simulink model "v2ggg2018"  (R2018b)
settings: Solver=VariableStepAuto  StartTime=0.0  StopTime=1  RelTol=1e-3
undefined symbols (not defined in the file): Ion, Lithium
libraries: powerlib x32, electricdrivelib x1, powerlib_meascontrol x1
settings Model: Creator=user  LastModifiedBy=utkar

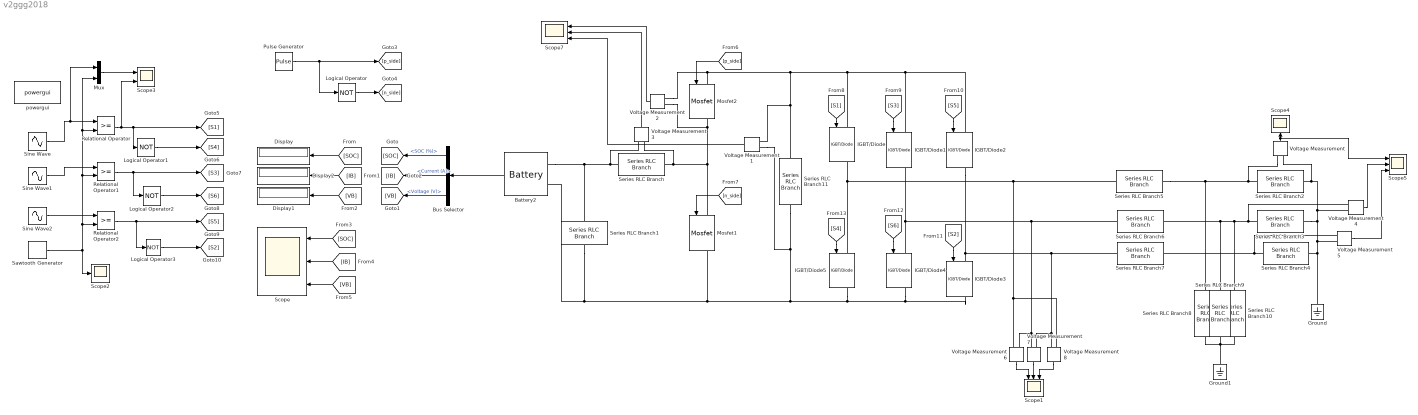
== system v2ggg2018 ==
  Battery2 : electricdrivelib/Extra Sources/Battery  BatType=Lithium-Ion  ShowTempParam=off  ThermalPreset=no  ShowAgeParam=off  NomV=24  NomQ=10  SOC=50  Batt_Tr=1e-4  PresetModel=on  MaxQ=10  MinV=18  FullV=27.9357  Dis_rate=4.3478  R=0.024  Normal_OP=9.0435  expZone="[25.9293     0.491304]"  current=[6.5 13 32.5]  Units=Time  Tci=20  NomT=20  T2=-30  MaxQ2=4.8  FullV2=7.1  Normal_OP2=5.655  expZone2="[6.58           1]"  Rca=0.6  ti=2000  Dp=0  Neq0=0  Tsim=1e6  Ta1=25  Qeol=5.4*0.9  Reol=0.013333*1.2  Char_age=[2.3478, 3]  Dis_age=[2.3478, 10]  N1=1500  N2=10500  N3=1000  N4=1400  Ta2=45  N5=950
  Bus Selector : BusSelector  OutputSignals=SOC (%),Current (A),Voltage (V)
  Display : Display
  Display1 : Display
  Display2 : Display
  Ground : powerlib/Elements/Ground  LConnTagsString=a
  Ground1 : powerlib/Elements/Ground  LConnTagsString=a
  IGBT/Diode{,1..5} (6 alike) : powerlib/Power Electronics/IGBT//Diode  Ron=1e-3  Rs=1e5  Cs=inf  Measurements=on
  Logical Operator{,1..3} (4 alike) : Logic  Operator=NOT  AllPortsSameDT=off  OutDataTypeStr=boolean
  Mosfet1 : powerlib/Power Electronics/Mosfet  Ron=0.1  Lon=0  Rd=0.01  Vfd=0  IC=0  Rs=1e5  Cs=inf  Measurements=on
  Mosfet2 : powerlib/Power Electronics/Mosfet  Ron=0.1  Lon=0  Rd=0.01  Vfd=0  IC=0  Rs=1e5  Cs=inf  Measurements=on
  Mux : Mux  Inputs=2
  Pulse Generator : DiscretePulseGenerator  PulseType=Time based  Period=1e-4  PulseWidth=40
  Relational Operator : RelationalOperator  OutDataTypeStr=boolean  RndMeth=Simplest
  Relational Operator1 : RelationalOperator  OutDataTypeStr=boolean  RndMeth=Simplest
  Relational Operator2 : RelationalOperator  OutDataTypeStr=boolean  RndMeth=Simplest
  Sawtooth Generator : powerlib_meascontrol/Pulse & Signal Generators/Sawtooth Generator  Freq=1e3  Phase=180  Ts=0
      settings: SourceProductName=Simscape Power Systems
  Scope{,1,5,7} (4 alike) : Scope  NumInputPorts=3
  Scope2 : Scope
  Scope3 : Scope  NumInputPorts=2
  Scope4 : Scope
  Series RLC Branch : powerlib/Elements/Series RLC Branch  LConnTagsString=__new0  RConnTagsString=__new0  BranchType=RL  Resistance=0.1  Inductance=1e-3  SetiL0=off  InitialCurrent=0  Capacitance=1e-6  Setx0=off  InitialVoltage=0  Measurements=None
  Series RLC Branch1 : powerlib/Elements/Series RLC Branch  LConnTagsString=__new0  RConnTagsString=__new0  BranchType=RC  Resistance=0.001  Inductance=1e-3  SetiL0=off  InitialCurrent=0  Capacitance=1000e-6  Setx0=off  InitialVoltage=0  Measurements=None
  Series RLC Branch10 : powerlib/Elements/Series RLC Branch  LConnTagsString=__new0  RConnTagsString=__new0  BranchType=C  Resistance=10  Inductance=1e-3  SetiL0=off  InitialCurrent=0  Capacitance=30e-6  Setx0=off  InitialVoltage=0  Measurements=None
  Series RLC Branch11 : powerlib/Elements/Series RLC Branch  LConnTagsString=__new0  RConnTagsString=__new0  BranchType=C  Resistance=10  Inductance=1e-3  SetiL0=off  InitialCurrent=0  Capacitance=5600e-6  Setx0=off  InitialVoltage=0  Measurements=None
  Series RLC Branch2 : powerlib/Elements/Series RLC Branch  LConnTagsString=__new0  RConnTagsString=__new0  BranchType=R  Resistance=10  Inductance=5e-3  SetiL0=off  InitialCurrent=0  Capacitance=1e-6  Setx0=off  InitialVoltage=0  Measurements=None
  Series RLC Branch3 : powerlib/Elements/Series RLC Branch  LConnTagsString=__new0  RConnTagsString=__new0  BranchType=R  Resistance=10  Inductance=5e-3  SetiL0=off  InitialCurrent=0  Capacitance=1e-6  Setx0=off  InitialVoltage=0  Measurements=None
  Series RLC Branch4 : powerlib/Elements/Series RLC Branch  LConnTagsString=__new0  RConnTagsString=__new0  BranchType=R  Resistance=10  Inductance=5e-3  SetiL0=off  InitialCurrent=0  Capacitance=1e-6  Setx0=off  InitialVoltage=0  Measurements=None
  Series RLC Branch5 : powerlib/Elements/Series RLC Branch  LConnTagsString=__new0  RConnTagsString=__new0  BranchType=L  Resistance=10  Inductance=5e-3  SetiL0=off  InitialCurrent=0  Capacitance=1e-6  Setx0=off  InitialVoltage=0  Measurements=None
  Series RLC Branch6 : powerlib/Elements/Series RLC Branch  LConnTagsString=__new0  RConnTagsString=__new0  BranchType=L  Resistance=10  Inductance=5e-3  SetiL0=off  InitialCurrent=0  Capacitance=1e-6  Setx0=off  InitialVoltage=0  Measurements=None
  Series RLC Branch7 : powerlib/Elements/Series RLC Branch  LConnTagsString=__new0  RConnTagsString=__new0  BranchType=L  Resistance=10  Inductance=5e-3  SetiL0=off  InitialCurrent=0  Capacitance=1e-6  Setx0=off  InitialVoltage=0  Measurements=None
  Series RLC Branch8 : powerlib/Elements/Series RLC Branch  LConnTagsString=__new0  RConnTagsString=__new0  BranchType=C  Resistance=10  Inductance=1e-3  SetiL0=off  InitialCurrent=0  Capacitance=30e-6  Setx0=off  InitialVoltage=0  Measurements=None
  Series RLC Branch9 : powerlib/Elements/Series RLC Branch  LConnTagsString=__new0  RConnTagsString=__new0  BranchType=C  Resistance=10  Inductance=1e-3  SetiL0=off  InitialCurrent=0  Capacitance=30e-6  Setx0=off  InitialVoltage=0  Measurements=None
  Sine Wave : Sin  Frequency=2*pi*50  SampleTime=0
  Sine Wave1 : Sin  Frequency=2*pi*50  Phase=2*pi/3  SampleTime=0
  Sine Wave2 : Sin  Frequency=2*pi*50  Phase=4*pi/3  SampleTime=0
  Voltage Measurement{,1..8} (9 alike) : powerlib/Measurements/Voltage Measurement  PhasorSimulation=off  OutputType=Complex  PSBequivalent=0
  powergui : powerlib/powergui  Priority=1  SimulationMode=Continuous  SampleTime=50e-6  frequency=60  Iterations=50  frequencyindice=0  Pbase=100e6  ErrMax=1e-4  UnitsV=kV  UnitsW=MW  buscounter=0  FunctionMessages=off  echomessages=off  EnableUseOfTLC=off  CurrentSourceSwitches=off  DisableSnubberDevices=off  DisableRonSwitches=off  DisableVfSwitches=off  DisplayEquations=off  SolverType=Tustin/Backward Euler (TBE)  Interpol=off  ExternalGateDelay=off  methode=off  Ts=100  x0status=blocks  SPID=on  SwTol=0  HookPort=off  RestoreLinks=warning  ResistiveCurrentMeasurement=off  Frange=[0:2:500]  Ylog=off  Xlog=on  ShowGrid=off  save=off  variable=ZData  structure=pasevol  ZoomFFT=off  StartTime=0.1  cycles=1  DisplayStyle=1  fundamental=50  FreqAxis=off  MaxFrequency=500  frequencyindicesteady=1  RmsSteady=1  display=off
  wires:
  Voltage Measurement3/1 -> Scope7/2
  [SOC] -> Scope/1
  [IB] -> Display2/1
  Bus Selector/2 -> [IB]  "<Current (A)>"
  Bus Selector/1 -> [SOC]  "<SOC (%)>"
  Logical Operator/1 -> [n_side]
  Bus Selector/3 -> [VB]  "<Voltage (V)>"
  [IB] -> Scope/2
  Battery2/1 -> Bus Selector/1
  Voltage Measurement2/1 -> Scope7/1
  [VB] -> Scope/3
  [VB] -> Display1/1
  Pulse Generator/1 -> Logical Operator/1, [p_side]
  [SOC] -> Display/1
  [p_side] -> Mosfet2/1
  [n_side] -> Mosfet1/1
  Voltage Measurement1/1 -> Scope7/3
  Voltage Measurement8/1 -> Scope1/3
  Voltage Measurement7/1 -> Scope1/2
  Voltage Measurement6/1 -> Scope1/1
  [S6] -> IGBT/Diode4/1
  Voltage Measurement5/1 -> Scope5/3
  Voltage Measurement4/1 -> Scope5/2
  Voltage Measurement/1 -> Scope5/1, Scope4/1
  [S4] -> IGBT/Diode5/1
  [S1] -> IGBT/Diode/1
  [S5] -> IGBT/Diode2/1
  [S3] -> IGBT/Diode1/1
  [S2] -> IGBT/Diode3/1
  Sine Wave1/1 -> Relational Operator1/1
  Relational Operator/1 -> Logical Operator1/1, [S1], Scope3/2
  Mux/1 -> Scope3/1
  Relational Operator2/1 -> Logical Operator3/1, [S5]
  Sawtooth Generator/1 -> Relational Operator1/2, Relational Operator/2, Mux/2, Relational Operator2/2, Scope2/1
  Logical Operator3/1 -> [S2]
  Logical Operator1/1 -> [S4]
  Sine Wave2/1 -> Relational Operator2/1
  Logical Operator2/1 -> [S6]
  Sine Wave/1 -> Mux/1, Relational Operator/1
  Relational Operator1/1 -> [S3], Logical Operator2/1
  connections:
  Mosfet2/RConn1 -- Voltage Measurement3/LConn1 -- Series RLC Branch/LConn1 -- Mosfet1/LConn1 -- Voltage Measurement2/LConn2
  Battery2/LConn1 -- Series RLC Branch1/LConn1 -- Voltage Measurement3/LConn2 -- Series RLC Branch/RConn1
  IGBT/Diode3/LConn1 -- Series RLC Branch7/LConn1 -- Voltage Measurement8/LConn1 -- Voltage Measurement7/LConn2 -- IGBT/Diode2/RConn1
  Voltage Measurement5/LConn2 -- Ground/LConn1 -- Series RLC Branch4/RConn1 -- Series RLC Branch3/RConn1 -- Voltage Measurement4/LConn2 -- Voltage Measurement/LConn2 -- Series RLC Branch2/RConn1
  Series RLC Branch1/RConn1 -- Battery2/LConn2 -- Mosfet1/RConn1 -- Series RLC Branch11/RConn1 -- Voltage Measurement1/LConn2 -- IGBT/Diode3/RConn1 -- IGBT/Diode4/RConn1 -- IGBT/Diode5/RConn1
  Voltage Measurement7/LConn1 -- Voltage Measurement6/LConn2 -- IGBT/Diode4/LConn1 -- IGBT/Diode1/RConn1 -- Series RLC Branch6/LConn1
  Voltage Measurement2/LConn1 -- Mosfet2/LConn1 -- Series RLC Branch11/LConn1 -- Voltage Measurement1/LConn1 -- IGBT/Diode/LConn1 -- IGBT/Diode1/LConn1 -- IGBT/Diode2/LConn1
  IGBT/Diode/RConn1 -- Voltage Measurement8/LConn2 -- Voltage Measurement6/LConn1 -- Series RLC Branch5/LConn1 -- IGBT/Diode5/LConn1
  Series RLC Branch3/LConn1 -- Voltage Measurement4/LConn1 -- Series RLC Branch10/LConn1 -- Series RLC Branch6/RConn1 -- Series RLC Branch9/LConn1
  Voltage Measurement5/LConn1 -- Series RLC Branch4/LConn1 -- Series RLC Branch7/RConn1
  Series RLC Branch5/RConn1 -- Series RLC Branch8/LConn1 -- Voltage Measurement/LConn1 -- Series RLC Branch2/LConn1
  Series RLC Branch8/RConn1 -- Series RLC Branch10/RConn1 -- Series RLC Branch9/RConn1 -- Ground1/LConn1
